simulink model "pmsmfoc_cleaned"  (R2022b)
settings: Solver=ode1  StartTime=0.0  StopTime=0.2  FixedStep=ctrlConst.TsSwitch  MaxStep=1e-6  RelTol=1e-3  EnableMultiTasking=on
PreLoadFcn:
  | %rtwdemo_pmsmfoc_data
StartFcn:
  | %clear executionProfile
StopFcn:
  | %try
  | %  AddExecutionProfileToDataInspector();
  | %end
undefined symbols (not defined in the file): ECM, EGM, fsw, g_msgCore0to2_pwmFrqSet, g_msgCore0to2_SpeedType_Switch, PWMFrqSwitch_C, SC_Ld_P, SC_Lq_P, SC_Psi_P, SC_Rs20_P, Ts_10ms, Ts_1ms, Tsw
libraries: MathLib x3
(part 1 of 2)
settings Model: Creator=The MathWorks, Inc.  LastModifiedBy=HP
settings SolverCC: AlgebraicLoopSolver=TrustRegion  InsertRTBMode=Never (minimum delay)
settings DataIOCC: LimitDataPoints=on  SaveFormat=Array  SaveOutput=off  SaveTime=off
settings OptimizationCC: DefaultParameterBehavior=Inlined  UseDivisionForNetSlopeComputation=on  UseFloatMulNetSlope=on  DefaultUnderspecifiedDataType=single  InlineInvariantSignals=on  PassReuseOutputArgsAs=Individual arguments  ExpressionDepthLimit=2147483647  ZeroExternalMemoryAtStartup=off  ZeroInternalMemoryAtStartup=off  NoFixptDivByZeroProtection=on  EfficientFloat2IntCast=on  LifeSpan=1  EfficientTunableParamExpr=on
settings DebuggingCC: ReadBeforeWriteMsg=DisableAll  WriteAfterWriteMsg=DisableAll  WriteAfterReadMsg=DisableAll  AlgebraicLoopMsg=none  MultiTaskDSMMsg=none  SingleTaskRateTransMsg=error  IntegerOverflowMsg=none  ParameterPrecisionLossMsg=none  BusObjectLabelMismatch=none  AssertControl=DisableAll  AllowSymbolicDim=off  StateNameClashWarn=warning  SFUnexpectedBacktrackingDiag=warning  SFNoUnconditionalDefaultTransitionDiag=warning  SFExecutionAtInitializationDiag=none  SFMachineParentedDataDiag=warning  IntegerSaturationMsg=none  UnitsInconsistencyMsg=none  ArithmeticOperatorsInVariantConditions=warning
settings HardwareCC: ProdBitPerPointer=32  ProdBitPerSizeT=32  ProdBitPerPtrDiffT=32  ProdLargestAtomicFloat=None  ProdWordSize=32  ProdHWDeviceType=Infineon->TriCore
settings ModelReferenceCC: UpdateModelReferenceTargets=IfOutOfDate  EnableRefExpFcnMdlSchedulingChecks=on  ModelReferenceNumInstancesAllowed=Single  PropagateSignalLabelsOutOfModel=off
settings SFSimCC: SFSimEcho=off  SimUseLocalCustomCode=off  SimGenImportedTypeDefs=on  MATLABDynamicMemAlloc=off  CustomCodeUndefinedFunction=UseInterfaceOnly
settings RTWCC: Description=Embedded Coder  SystemTargetFile=ert.tlc  GenCodeOnly=on  GenerateMakefile=off  TemplateMakefile=ec_target.tmf  RTWVerbose=off  RTWUseLocalCustomCode=off  CodeExecutionProfiling=on  CodeProfilingSaveOptions=AllData  CodeProfilingInstrumentation=detailed
settings CodeAppCC: ForceParamTrailComments=on  IgnoreCustomStorageClasses=off  IgnoreTestpoints=on  MaxIdLength=64  SimulinkDataObjDesc=on  MATLABFcnDesc=on  CustomSymbolStrGlobalVar=GR$N$M  CustomSymbolStrType=pmsmfoc_$N$M  CustomSymbolStrFcn=$N$M$F  CustomSymbolStrFcnArg=$I$N$M  CustomSymbolStrMacro=$N$M  InsertBlockDesc=on  StateflowObjectComments=on  MATLABSourceComments=on  InternalIdentifier=Classic
settings ERTTargetCC: TargetLangStandard=C99 (ISO)  UtilityFuncGeneration=Shared location  MultiwordLength=2048  CombineSignalStateStructs=on  SupportAbsoluteTime=off  SupportNonFinite=off  SupportComplex=off  SupportNonInlinedSFcns=on  RemoveResetFunc=off  ParenthesesLevel=Maximum  GenerateASAP2=on  InlinedParameterPlacement=NonHierarchical  ERTCustomFileTemplate=example_file_process.tlc  EnableDataOwnership=on  ConvertIfToSwitch=off  SuppressUnreachableDefaultCases=off  MemSecPackage=Simulink  MemSecDataConstants=MemConst  MemSecDataParameters=MemConstVolatile
settings ConfigComp: CovMetricSettings=dcmtrzow  CovHTMLOptions=-aTS=1 -bRG=1 -bTC=1 -hTR=0 -nFC=0 -scm=1 -bcm=1 -xEv=0  CovSaveCumulativeToWorkspaceVar=on  CovSaveSingleToWorkspaceVar=on  CovExternalEMLEnable=off  CovSFcnEnable=off
settings SimscapeCC: SimscapeNormalizeSystem=off

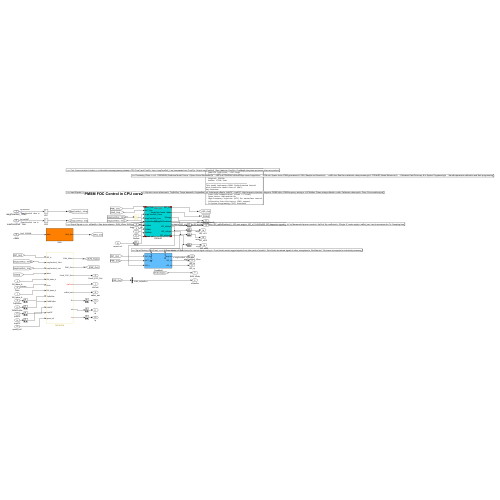
[thumbnail: Simulink's stored preview of the top-level diagram]
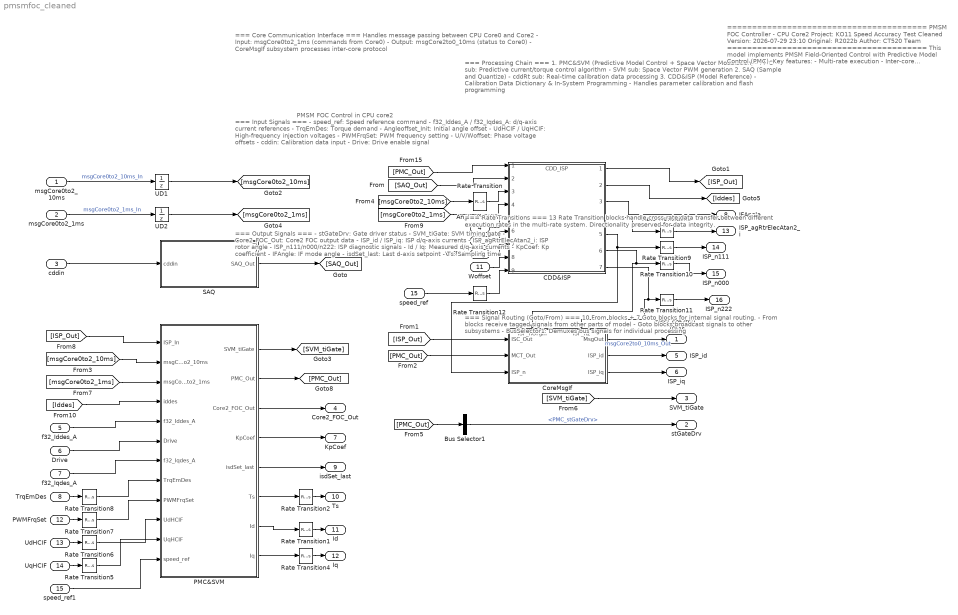
== system pmsmfoc_cleaned ==
  note: PMSM FOC Control in CPU core2
  note: === Core Communication Interface ===\nHandles message passing between CPU Core0 and Core2\n- Input: msgCore0to2_1ms (commands from Core0)\n- Output: msgCore2to0_10ms (status to Core0)\n- CoreMsgIf subsystem processes inter-core protocol
  note: === Input Signals ===\n- speed_ref: Speed reference command\n- f32_Iddes_A / f32_Iqdes_A: d/q-axis current references\n- TrqEmDes: Torque demand\n- Angleoffset_Init: Initial angle offset\n- UdHCIF / UqHCIF: High-frequency injection voltages\n- PWMFrqSet: PWM frequency setting\n- U/V/Woffset: Phase voltage offsets\n- cddin: Calibration data input\n- Drive: Drive enable signal
  note: === Output Signals ===\n- stGateDrv: Gate driver status\n- SVM_tiGate: SVM timing gate\n- Core2_FOC_Out: Core2 FOC output data\n- ISP_id / ISP_iq: ISP d/q-axis currents\n- ISP_agRtrElecAtan2_i: ISP rotor angle\n- ISP_n111/n000/n222: ISP diagnostic signals\n- Id / Iq: Measured d/q-axis currents\n- KpCoef: Kp coefficient\n- IFAngle: IF mode angle\n- isdSet_last: Last d-axis setpoint\n- Ts: Sampling time
  note: === Processing Chain ===\n1. PMC&SVM (Predictive Model Control + Space Vector Modulation)\n - PMC sub: Predictive current/torque control algorithm\n - SVM sub: Space Vector PWM generation\n2. SAQ (Sample and Quantize)\n - cddRt sub: Real-time calibration data processing\n3. CDD&ISP (Model Reference)\n - Calibration Data Dictionary & In-System Programming\n - Handles parameter calibration and flash programming
  note: === Rate Transitions ===\n13 Rate Transition blocks handle cross-rate data transfer\nbetween different execution rates in the multi-rate system.\nDirectionality preserved for data integrity.
  note: === Signal Routing (Goto/From) ===\n10 From blocks + 7 Goto blocks for internal signal routing.\n- From blocks receive tagged signals from other parts of model\n- Goto blocks broadcast signals to other subsystems\n- BusSelector1: Demuxes bus signals for individual processing
  note: ========================================
      |   PMSM FOC Controller - CPU Core2
      |   Project: KO11 Speed Accuracy Test
      |   Cleaned Version: 2026-07-29 23:10
      |   Original: R2022b
      |   Author: CT520 Team
      | ========================================
      | This model implements PMSM Field-Oriented Control
      | with Predictive Model Control (PMC).
      | Key features:
      | - Multi-rate execution
      | - Inter-core communication (Core0 <-> Core2)
      | - Space Vector PWM modulation
      | - High-Frequency Injection (HFI) for sensorless control
      | - Calibration Data Dictionary (CDD) support
      | - In-System Programming (ISP) interface
  msgCore0to2_10ms : Inport  OutDataTypeStr=Bus: Sig10ms02ST  SampleTime=Ts_1ms  BusOutputAsStruct=on
  msgCore0to2_1ms : Inport  Port=2  OutDataTypeStr=Bus: Sig1ms02ST  SampleTime=Ts_1ms  BusOutputAsStruct=on
  cddin : Inport  Port=3  OutDataTypeStr=Bus: Core2_CDDIN2  SampleTime=Tsw  BusOutputAsStruct=on
  Angleoffset_Init : Inport  Port=4  OutDataTypeStr=int16  SampleTime=Ts_10ms
  f32_Iddes_A : Inport  Port=5
  Drive : Inport  Port=6  OutDataTypeStr=boolean
  f32_Iqdes_A : Inport  Port=7
  TrqEmDes : Inport  Port=8
  Uoffset : Inport  Port=9
  Voffset : Inport  Port=10
  Woffset : Inport  Port=11
  PWMFrqSet : Inport  Port=12
  UdHCIF : Inport  Port=13
  UqHCIF : Inport  Port=14
  speed_ref : Inport  Port=15
  Bus Selector1 : BusSelector  OutputSignals=PMC_stGateDrv
  CDD&ISP : ModelReference  ModelNameDialog=CDD_ISP.slx  SimulationMode=Normal  ModelReferenceVersion=1.237
  CoreMsgIf : Subsystem
      settings: PortSchema="{\"entries\":[{\"content\":{\"sides\":[{\"content\":{\"connectorIds\":[\"In1\",\"In2\",\"In3\"]},\"type\":\"ConnectorPlacement.EquallySpacedRectSide\",\"uuid\":\"1bc9449b-5392-4ed5-810c-ef0b1f3a3873\"},{\"content\":{\"connectorIds\":[\"Out1\",\"Out2\",\"Out3\"],\"side\":\"RIGHT\"},\"type\":\"ConnectorPlacement.EquallySpacedRectSide\",\"uuid\":\"ebce0c42-110a-49f6-97c9-7794c95f763f\"},{\"content\":{\"connectorIds\":[\"In4\",\"In5\"],\"side\":\"TOP\"},\"type\":\"ConnectorPlacement.EquallySpacedRectSide\",\"uuid\":\"d14212b0-cf9d-44fe-a2d1-1375008f2372\"}]},\"type\":\"ConnectorPlacement.EquallySpacedConnector\",\"uuid\":\"c8a2bb93-ddbf-4abc-bd38-97ecc81d6200\"}],\"packageUris\":[\"http://schema.mathworks.com/mf0/Connector/R2020b\"],\"version\":\"1.0\"}"
  PMC&SVM : Subsystem  RequirementInfo={} %GIDa_aba5f94c_bdce_4442_83f7_df5d7516f2fa
      settings: MinAlgLoopOccurrences=on
  Rate Transition : RateTransition  Deterministic=off
  Rate Transition{1..2,4..8,12} (8 alike) : RateTransition  Deterministic=off  InitialCondition=ECM.Init
  Rate Transition{3,9..11} (4 alike) : RateTransition
  SAQ : Subsystem
  UD1 : UnitDelay  SampleTime=-1  HasFrameUpgradeWarning=on
  UD2 : UnitDelay  SampleTime=-1  HasFrameUpgradeWarning=on
  speed_ref1 : InportShadow  Port=15
  msgCore2to0_10ms : Outport  OutDataTypeStr=Bus: Sig10ms20ST  VectorParamsAs1DForOutWhenUnconnected=off
  stGateDrv : Outport  Port=2  VectorParamsAs1DForOutWhenUnconnected=off
  SVM_tiGate : Outport  Port=3  VectorParamsAs1DForOutWhenUnconnected=off
  Core2_FOC_Out : Outport  Port=4
  ISP_id : Outport  Port=5
  ISP_iq : Outport  Port=6
  KpCoef : Outport  Port=7
  IFAngle : Outport  Port=8
  isdSet_last : Outport  Port=9
  Ts : Outport  Port=10
  Id : Outport  Port=11
  Iq : Outport  Port=12
  ISP_agRtrElecAtan2_i : Outport  Port=13
  ISP_n111 : Outport  Port=14  OutDataTypeStr=single
  ISP_n000 : Outport  Port=15  OutDataTypeStr=single
  ISP_n222 : Outport  Port=16  OutDataTypeStr=single
  wires:
  cddin/1 -> SAQ/1(cddin)
  SAQ/1(SAQ_Out) -> [SAQ_Out]
  [SAQ_Out] -> CDD&ISP/2
  CDD&ISP/1 -> [ISP_Out]
  [ISP_Out] -> PMC&SVM/1(ISP_In)
  [PMC_Out] -> CDD&ISP/1
  Bus Selector1/1 -> stGateDrv/1  "<PMC_stGateDrv>"
  [msgCore0to2_10ms] -> PMC&SVM/2(msgCore0to2_10ms)
  msgCore0to2_1ms/1 -> UD2/1  "msgCore0to2_1ms_In"
  [msgCore0to2_10ms] -> Rate Transition/1
  [ISP_Out] -> CoreMsgIf/1(ISC_Out)
  [PMC_Out] -> CoreMsgIf/2(MCT_Out)
  [PMC_Out] -> Bus Selector1/1
  [SVM_tiGate] -> SVM_tiGate/1
  CoreMsgIf/1(MsgOut) -> msgCore2to0_10ms/1  "msgCore2to0_10ms_Out"
  msgCore0to2_10ms/1 -> UD1/1  "msgCore0to2_10ms_In"
  UD1/1 -> [msgCore0to2_10ms]
  [msgCore0to2_1ms] -> PMC&SVM/3(msgCore0to2_1ms)
  UD2/1 -> [msgCore0to2_1ms]
  [msgCore0to2_1ms] -> CDD&ISP/4
  PMC&SVM/1(SVM_tiGate) -> [SVM_tiGate]
  PMC&SVM/2(PMC_Out) -> [PMC_Out]
  Rate Transition/1 -> CDD&ISP/3
  PMC&SVM/3(Core2_FOC_Out) -> Core2_FOC_Out/1
  CoreMsgIf/2(ISP_id) -> ISP_id/1
  CoreMsgIf/3(ISP_iq) -> ISP_iq/1
  CDD&ISP/2 -> [Iddes]
  [Iddes] -> PMC&SVM/4(iddes)
  Angleoffset_Init/1 -> CDD&ISP/5
  f32_Iddes_A/1 -> PMC&SVM/5(f32_Iddes_A)
  Drive/1 -> PMC&SVM/6(Drive)
  f32_Iqdes_A/1 -> PMC&SVM/7(f32_Iqdes_A)
  PMC&SVM/4(KpCoef) -> KpCoef/1
  TrqEmDes/1 -> Rate Transition8/1
  PMC&SVM/5(isdSet_last) -> isdSet_last/1
  PMC&SVM/6(Ts) -> Rate Transition2/1
  PMC&SVM/7(Id) -> Rate Transition1/1
  PMC&SVM/8(Iq) -> Rate Transition4/1
  Uoffset/1 -> CDD&ISP/6
  Voffset/1 -> CDD&ISP/7
  Woffset/1 -> CDD&ISP/8
  PWMFrqSet/1 -> Rate Transition7/1
  Rate Transition4/1 -> Iq/1
  Rate Transition1/1 -> Id/1
  Rate Transition2/1 -> Ts/1
  UdHCIF/1 -> Rate Transition6/1
  UqHCIF/1 -> Rate Transition5/1
  CDD&ISP/3 -> IFAngle/1
  CDD&ISP/4 -> Rate Transition3/1
  Rate Transition3/1 -> ISP_agRtrElecAtan2_i/1
  Rate Transition5/1 -> PMC&SVM/11(UqHCIF)
  Rate Transition6/1 -> PMC&SVM/10(UdHCIF)
  Rate Transition7/1 -> PMC&SVM/9(PWMFrqSet)
  Rate Transition8/1 -> PMC&SVM/8(TrqEmDes)
  CDD&ISP/5 -> Rate Transition9/1, CoreMsgIf/3(ISP_n)
  Rate Transition9/1 -> ISP_n111/1
  CDD&ISP/6 -> Rate Transition10/1, CoreMsgIf/4(ISP_nOrgin)
  Rate Transition10/1 -> ISP_n000/1
  speed_ref/1 -> Rate Transition12/1
  Rate Transition12/1 -> CDD&ISP/9
  Rate Transition11/1 -> ISP_n222/1
  CDD&ISP/7 -> Rate Transition11/1, CoreMsgIf/5(ISP_n2)
  speed_ref1/1 -> PMC&SVM/12(speed_ref)

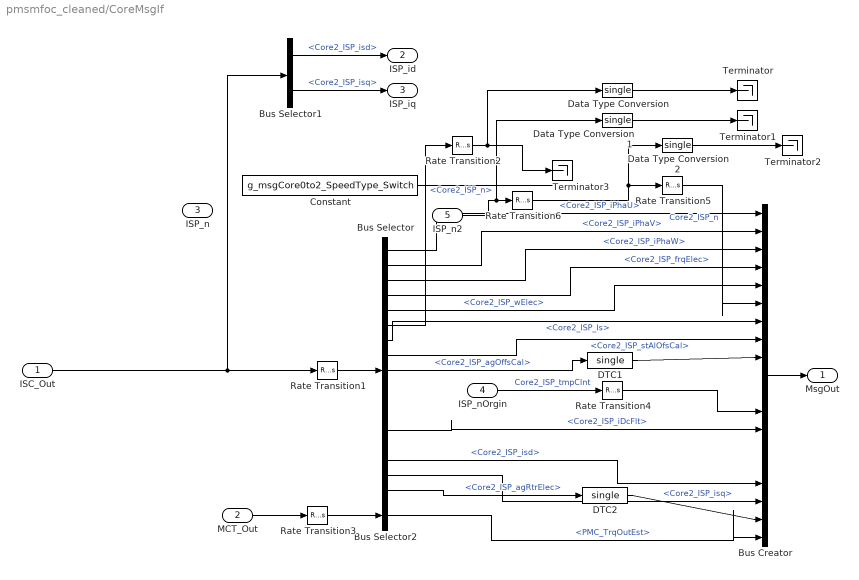
== system pmsmfoc_cleaned/CoreMsgIf ==
  ISC_Out : Inport  OutDataTypeStr=Bus: Core2_ISP_Out
  MCT_Out : Inport  Port=2
  ISP_n : Inport  Port=3
  ISP_nOrgin : Inport  Port=4
  ISP_n2 : Inport  Port=5
  Bus Creator : BusCreator  Inputs=19  OutDataTypeStr=Bus:Sig10ms20ST  NonVirtualBus=on
      settings: InheritFromInputs=off
  Bus Selector : BusSelector  OutputSignals=Core2_ISP_AnaOut.Core2_ISP_iPhabc.Core2_ISP_iPhaU,Core2_ISP_AnaOut.Core2_ISP_iPhabc.Core2_ISP_iPhaV,Core2_ISP_AnaOut.Core2_ISP_iPhabc.Core2_ISP_iPhaW,Core2_ISP_nx.Core2_ISP_frqElec,Core2_ISP_nx.Core2_ISP_wElec,Core2_ISP_nx.Core2_ISP_n,Core2_ISP_Isx.Core2_ISP_Is,Core2_ISP_nx.Core2_ISP_stAlOfsCal,Core2_ISP_nx.Core2_ISP_agOffsCal,Core2_ISC_tmpOut.Core2_ISP_tmpMaxIGBT,Core2_ISC_tmpOut.Core2_ISP_tmpClnt,Core2_ISC_tmpOut.Core2_ISP_lossTotalIGBT,Core2_ISC_tmpOut.Core2_ISP_iDcFlt,Core2_ISP_AnaOut.Core2_ISP_bIphCalDone,Core2_ISP_Isx.Core2_ISP_isd,Core2_ISP_Isx.Core2_ISP_isq,Core2_ISP_nx.Core2_ISP_agRtrElec
  Bus Selector1 : BusSelector  OutputSignals=Core2_ISP_Isx.Core2_ISP_isd,Core2_ISP_Isx.Core2_ISP_isq
  Bus Selector2 : BusSelector  OutputSignals=PMC_TrqOutEst
  Constant : Constant  Value=g_msgCore0to2_SpeedType_Switch
  DTC1 : DataTypeConversion  OutDataTypeStr=single  SaturateOnIntegerOverflow=off  RndMeth=Floor
  DTC2 : DataTypeConversion  OutDataTypeStr=single  SaturateOnIntegerOverflow=off  RndMeth=Floor
  Data Type Conversion : DataTypeConversion  OutDataTypeStr=single  SaturateOnIntegerOverflow=off  RndMeth=Floor
  Data Type Conversion1 : DataTypeConversion  OutDataTypeStr=single  SaturateOnIntegerOverflow=off  RndMeth=Floor
  Data Type Conversion2 : DataTypeConversion  OutDataTypeStr=single  SaturateOnIntegerOverflow=off  RndMeth=Floor
  Rate Transition{1..6} (6 alike) : RateTransition  Deterministic=off  OutPortSampleTime=Ts_1ms
  Terminator{,1..3} (4 alike) : Terminator
  MsgOut : Outport  OutDataTypeStr=Bus: Sig10ms20ST  VectorParamsAs1DForOutWhenUnconnected=off
  ISP_id : Outport  Port=2
  ISP_iq : Outport  Port=3
  wires:
  MCT_Out/1 -> Rate Transition3/1
  Rate Transition3/1 -> Bus Selector2/1
  Bus Selector/13 -> Bus Creator/13  "<Core2_ISP_iDcFlt>"
  ISC_Out/1 -> Rate Transition1/1, Bus Selector1/1
  Rate Transition1/1 -> Bus Selector/1
  Bus Selector/5 -> Bus Creator/5  "<Core2_ISP_wElec>"
  Bus Selector/4 -> Bus Creator/4  "<Core2_ISP_frqElec>"
  Bus Creator/1 -> MsgOut/1
  Bus Selector/7 -> Bus Creator/7  "<Core2_ISP_Is>"
  Bus Selector/8 -> Bus Creator/8  "<Core2_ISP_stAlOfsCal>"
  Bus Selector/9 -> DTC1/1  "<Core2_ISP_agOffsCal>"
  DTC1/1 -> Bus Creator/9
  Bus Selector/17 -> DTC2/1  "<Core2_ISP_agRtrElec>"
  Bus Selector/16 -> Bus Creator/17  "<Core2_ISP_isq>"
  Bus Selector/15 -> Bus Creator/16  "<Core2_ISP_isd>"
  DTC2/1 -> Bus Creator/18
  Bus Selector2/1 -> Bus Creator/19  "<PMC_TrqOutEst>"
  Bus Selector1/1 -> ISP_id/1  "<Core2_ISP_isd>"
  Bus Selector1/2 -> ISP_iq/1  "<Core2_ISP_isq>"
  Bus Selector/3 -> Bus Creator/3  "<Core2_ISP_iPhaW>"
  Bus Selector/2 -> Bus Creator/2  "<Core2_ISP_iPhaV>"
  Bus Selector/1 -> Bus Creator/1  "<Core2_ISP_iPhaU>"
  Rate Transition4/1 -> Bus Creator/12
  ISP_nOrgin/1 -> Rate Transition4/1  "Core2_ISP_tmpClnt"
  Bus Selector/6 -> Rate Transition2/1  "<Core2_ISP_n>"
  Rate Transition6/1 -> Data Type Conversion2/1, Rate Transition5/1
  ISP_n2/1 -> Data Type Conversion1/1, Rate Transition6/1
  Constant/1 -> ?
  Rate Transition2/1 -> Terminator3/1, Data Type Conversion/1
  Rate Transition5/1 -> Bus Creator/6  "Core2_ISP_n"
  Data Type Conversion/1 -> Terminator/1
  Data Type Conversion1/1 -> Terminator1/1
  Data Type Conversion2/1 -> Terminator2/1

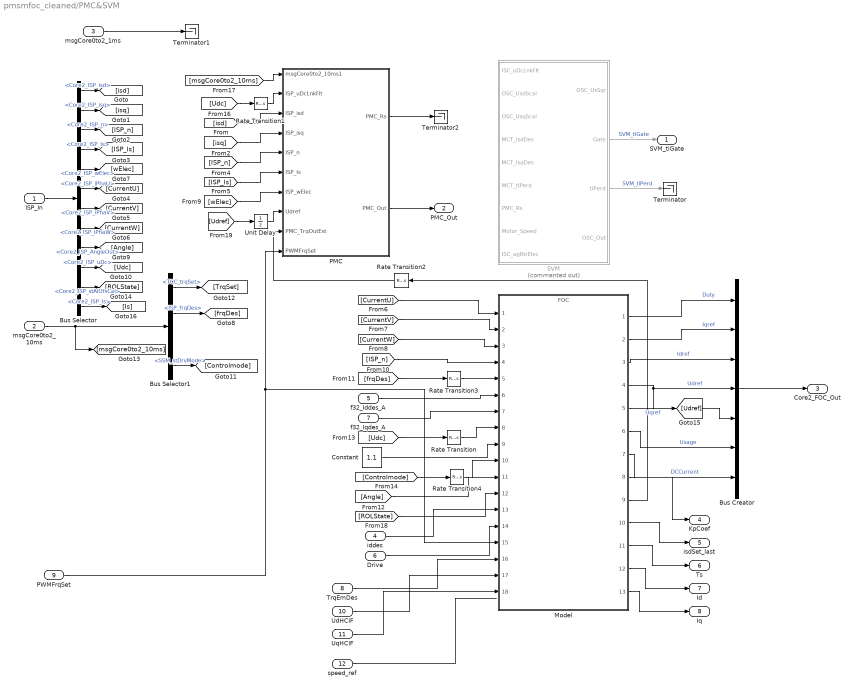
== system pmsmfoc_cleaned/PMC&SVM ==
  ISP_In : Inport  RequirementInfo={} %GIDa_f6540206_9371_47ef_bcdb_2ea40a07804d
  msgCore0to2_10ms : Inport  RequirementInfo={} %GIDa_db689c64_39e8_4f82_8312_263842f9e924  Port=2
  msgCore0to2_1ms : Inport  Port=3
  iddes : Inport  Port=4
  f32_Iddes_A : Inport  Port=5
  Drive : Inport  Port=6
  f32_Iqdes_A : Inport  Port=7
  TrqEmDes : Inport  Port=8
  PWMFrqSet : Inport  Port=9
  UdHCIF : Inport  Port=10
  UqHCIF : Inport  Port=11
  speed_ref : Inport  Port=12
  Bus Creator : BusCreator  Inputs=7  OutDataTypeStr=Bus: Core2_FOC_Out  NonVirtualBus=on
  Bus Selector : BusSelector  OutputSignals=Core2_ISP_Isx.Core2_ISP_isd,Core2_ISP_Isx.Core2_ISP_isq,Core2_ISP_nx.Core2_ISP_n,Core2_ISP_Isx.Core2_ISP_Is,Core2_ISP_nx.Core2_ISP_wElec,Core2_ISP_AnaOut.Core2_ISP_iPhabc.Core2_ISP_iPhaU,Core2_ISP_AnaOut.Core2_ISP_iPhabc.Core2_ISP_iPhaV,Core2_ISP_AnaOut.Core2_ISP_iPhabc.Core2_ISP_iPhaW,Core2_ISP_Isx.Core2_ISP_AngleOut,Core2_ISP_AnaOut.Core2_ISP_uDc,Core2_ISP_nx.Core2_ISP_stAlOfsCal,Core2_ISP_Isx.Core2_ISP_Is
  Bus Selector1 : BusSelector  OutputSignals=TCC_trqSet,ISP_frqDes,ISP_isDes,SSM_stDrvMode
  Constant : Constant  Value=1.1  OutDataTypeStr=single
  Model : ModelReference  ModelNameDialog=FOC.slx  SimulationMode=Normal  ModelReferenceVersion=1.230
  PMC : Subsystem  RequirementInfo={} %GIDa_45aea5b4_73b0_47d7_923a_5575377c0528  SystemSampleTime=Tsw
  Rate Transition{,1..3} (4 alike) : RateTransition  Deterministic=off
  Rate Transition4 : RateTransition  Deterministic=off  InitialCondition=ECM.Init
  SVM : Subsystem  Commented=on
  Terminator : Terminator
  Terminator1 : Terminator
  Terminator2 : Terminator
  Unit Delay : UnitDelay  SampleTime=-1  HasFrameUpgradeWarning=on
  SVM_tiGate : Outport  RequirementInfo={} %GIDa_247e6739_f09d_406d_b522_add8602f32ed  VectorParamsAs1DForOutWhenUnconnected=off
  PMC_Out : Outport  Port=2  OutDataTypeStr=Bus: Core2_PMC_Out  VectorParamsAs1DForOutWhenUnconnected=off
  Core2_FOC_Out : Outport  Port=3
  KpCoef : Outport  Port=4
  isdSet_last : Outport  Port=5
  Ts : Outport  Port=6
  Id : Outport  Port=7
  Iq : Outport  Port=8
  wires:
  SVM/2(Gate) -> SVM_tiGate/1  "SVM_tiGate"
  Rate Transition1/1 -> PMC/2(ISP_uDcLnkFlt)
  ISP_In/1 -> Bus Selector/1
  PMC/2(PMC_Out) -> PMC_Out/1
  msgCore0to2_10ms/1 -> Bus Selector1/1, [msgCore0to2_10ms]
  SVM/3(tiPerd) -> Terminator/1  "SVM_tiPerd"
  msgCore0to2_1ms/1 -> Terminator1/1
  PMC/1(PMC_Rs) -> Terminator2/1
  Constant/1 -> Model/9
  Rate Transition3/1 -> Model/5
  Rate Transition/1 -> Model/8
  Rate Transition4/1 -> Model/10
  Model/1 -> Bus Creator/1  "Duty"
  Model/2 -> Bus Creator/2  "Iqref"
  Model/3 -> Bus Creator/3  "Idref"
  Model/4 -> Bus Creator/4, [Udref]  "Udref"
  Model/5 -> Bus Creator/5  "Uqref"
  Bus Creator/1 -> Core2_FOC_Out/1
  Bus Selector/1 -> [isd]  "<Core2_ISP_isd>"
  [isd] -> PMC/3(ISP_isd)
  [isq] -> PMC/4(ISP_isq)
  Bus Selector/2 -> [isq]  "<Core2_ISP_isq>"
  Bus Selector/3 -> [ISP_n]  "<Core2_ISP_n>"
  [ISP_n] -> PMC/5(ISP_n)
  Bus Selector/4 -> [ISP_Is]  "<Core2_ISP_Is>"
  [ISP_Is] -> PMC/6(ISP_Is)
  Bus Selector/6 -> [CurrentU]  "<Core2_ISP_iPhaU>"
  Bus Selector/7 -> [CurrentV]  "<Core2_ISP_iPhaV>"
  Bus Selector/8 -> [CurrentW]  "<Core2_ISP_iPhaW>"
  [CurrentU] -> Model/1
  [CurrentV] -> Model/2
  [CurrentW] -> Model/3
  Bus Selector/5 -> [wElec]  "<Core2_ISP_wElec>"
  [wElec] -> PMC/7(ISP_wElec)
  [ISP_n] -> Model/4
  Bus Selector1/2 -> [frqDes]  "<ISP_frqDes>"
  [frqDes] -> Rate Transition3/1
  Bus Selector/9 -> [Angle]  "<Core2_ISP_AngleOut>"
  [Angle] -> Model/11
  Bus Selector/10 -> [Udc]  "<Core2_ISP_uDc>"
  [Udc] -> Rate Transition/1
  Bus Selector1/4 -> [Controlmode]  "<SSM_stDrvMode>"
  [Controlmode] -> Rate Transition4/1
  Bus Selector1/1 -> [TrqSet]  "<TCC_trqSet>"
  [Udc] -> Rate Transition1/1
  [msgCore0to2_10ms] -> PMC/1(msgCore0to2_10ms1)
  Bus Selector/11 -> [ROLState]  "<Core2_ISP_stAlOfsCal>"
  [ROLState] -> Model/12
  iddes/1 -> Model/13
  f32_Iddes_A/1 -> Model/6
  Drive/1 -> Model/14
  f32_Iqdes_A/1 -> Model/7
  [Udref] -> Unit Delay/1
  Unit Delay/1 -> PMC/8(Udref)
  Bus Selector/12 -> [Is]  "<Core2_ISP_Is>"
  Model/8 -> KpCoef/1
  Model/6 -> Bus Creator/6  "Usage"
  Model/7 -> Bus Creator/7  "DCCurrent"
  Model/9 -> Rate Transition2/1
  TrqEmDes/1 -> Model/16
  Model/10 -> isdSet_last/1
  Model/11 -> Ts/1
  Model/12 -> Id/1
  Model/13 -> Iq/1
  PWMFrqSet/1 -> PMC/10(PWMFrqSet), Model/15
  UdHCIF/1 -> Model/17
  UqHCIF/1 -> Model/18
  Rate Transition2/1 -> PMC/9(PMC_TrqOutEst)
  speed_ref/1 -> ?

== system pmsmfoc_cleaned/SAQ ==
  cddin : Inport
  cddRt : Subsystem
  SAQ_Out : Outport  OutDataTypeStr=Bus: Core2_SAQ_Out  VectorParamsAs1DForOutWhenUnconnected=off
      settings: AttributesFormatString=Disable Action: %<OutputWhenDisabled>
  wires:
  cddRt/1(cddSig) -> SAQ_Out/1  "cddRt"
  cddin/1 -> cddRt/1(cddSt)

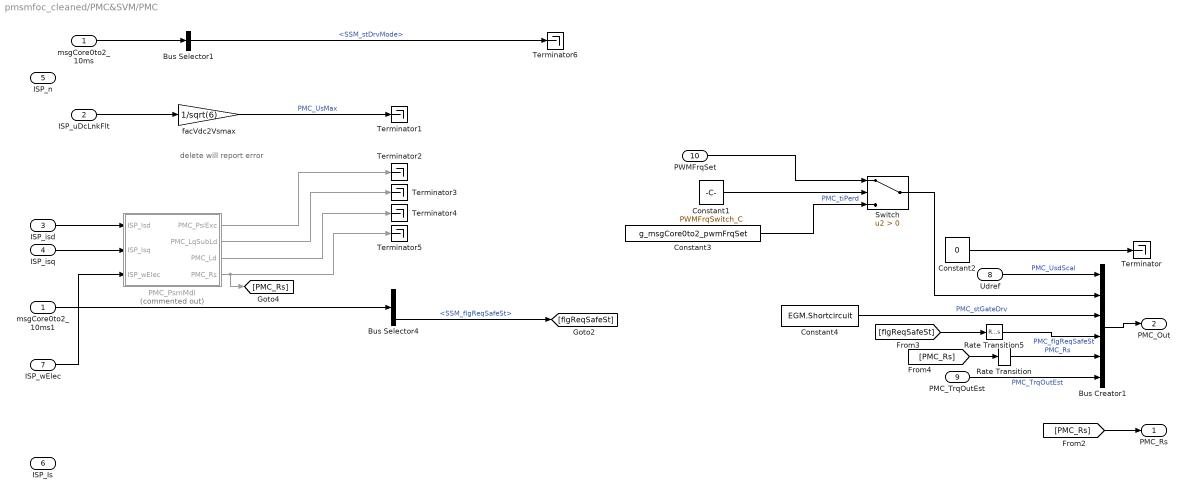
== system pmsmfoc_cleaned/PMC&SVM/PMC ==
  note: delete will report error
  msgCore0to2_10ms1 : Inport  RequirementInfo={} %GIDa_62968669_2ac2_4296_9b34_9acab11e3351
  ISP_uDcLnkFlt : Inport  RequirementInfo={} %GIDa_ca93117e_11ed_4a5d_b591_b702703c2b5a  Port=2
  ISP_isd : Inport  RequirementInfo={} %GIDa_4c76f347_a6a1_47a4_b7d0_60bec3ffd976  Port=3
  ISP_isq : Inport  RequirementInfo={} %GIDa_70459766_063a_410f_849e_470931a9729a  Port=4
  ISP_n : Inport  Port=5
  ISP_Is : Inport  Port=6
  ISP_wElec : Inport  RequirementInfo={} %GIDa_15028701_01af_406d_8077_8bad37e851e9  Port=7
  Udref : Inport  Port=8
  PMC_TrqOutEst : Inport  Port=9
  PWMFrqSet : Inport  Port=10
  Bus Creator1 : BusCreator  Inputs=6  OutDataTypeStr=Bus: Core2_PMC_Out  NonVirtualBus=on
  Bus Selector1 : BusSelector  OutputSignals=SSM_stDrvMode
  Bus Selector4 : BusSelector  OutputSignals=SSM_stGateDrv,SSM_stDrvMode,SSM_flgReqSafeSt
  Constant1 : Constant  Value=PWMFrqSwitch_C
  Constant2 : Constant  Value=0  OutDataTypeStr=single  SampleTime=-1
  Constant3 : Constant  Value=g_msgCore0to2_pwmFrqSet  OutDataTypeStr=single  SampleTime=-1
  Constant4 : Constant  Value=EGM.Shortcircuit  OutDataTypeStr=Enum: EGM
  PMC_PsmMdl : Subsystem  RequirementInfo={} %GIDa_c46a785d_0a8b_4cc8_8d66_3e5f2fce2378  Commented=on
  Rate Transition : RateTransition  Deterministic=off
  Rate Transition5 : RateTransition  Deterministic=off  OutPortSampleTime=Tsw
  Switch : Switch  Criteria=u2 > Threshold  SaturateOnIntegerOverflow=off  InputSameDT=off
  Terminator{,1..6} (7 alike) : Terminator
  facVdc2Vsmax : Gain  RequirementInfo={} %GIDa_223ddcfe_885a_4a4c_9204_a9c8c9b1baab  Gain=1/sqrt(6)
  msgCore0to2_10ms : InportShadow
  PMC_Rs : Outport  VectorParamsAs1DForOutWhenUnconnected=off
  PMC_Out : Outport  Port=2  OutDataTypeStr=Bus: Core2_PMC_Out  VectorParamsAs1DForOutWhenUnconnected=off
  wires:
  Constant2/1 -> Terminator/1
  Udref/1 -> Bus Creator1/1  "PMC_UsdScal"
  facVdc2Vsmax/1 -> Terminator1/1  "PMC_UsMax"
  ISP_wElec/1 -> PMC_PsmMdl/3(ISP_wElec)
  ISP_uDcLnkFlt/1 -> facVdc2Vsmax/1
  PMC_PsmMdl/3(PMC_Ld) -> Terminator4/1
  PMC_PsmMdl/2(PMC_LqSubLd) -> Terminator3/1
  PMC_PsmMdl/1(PMC_PsiExc) -> Terminator2/1
  msgCore0to2_10ms1/1 -> Bus Selector4/1
  ISP_isq/1 -> PMC_PsmMdl/2(ISP_Isq)
  ISP_isd/1 -> PMC_PsmMdl/1(ISP_Isd)
  Bus Creator1/1 -> PMC_Out/1
  Constant4/1 -> Bus Creator1/3  "PMC_stGateDrv"
  Bus Selector4/3 -> [flgReqSafeSt]  "<SSM_flgReqSafeSt>"
  Rate Transition5/1 -> Bus Creator1/4  "PMC_flgReqSafeSt"
  Constant3/1 -> Switch/3  "PMC_tiPerd"
  PMC_PsmMdl/4(PMC_Rs) -> Terminator5/1, [PMC_Rs]
  [flgReqSafeSt] -> Rate Transition5/1
  [PMC_Rs] -> Rate Transition/1
  msgCore0to2_10ms/1 -> Bus Selector1/1
  Bus Selector1/1 -> Terminator6/1  "<SSM_stDrvMode>"
  [PMC_Rs] -> PMC_Rs/1
  Rate Transition/1 -> Bus Creator1/5  "PMC_Rs"
  PMC_TrqOutEst/1 -> Bus Creator1/6  "PMC_TrqOutEst"
  Constant1/1 -> Switch/2
  PWMFrqSet/1 -> Switch/1
  Switch/1 -> Bus Creator1/2

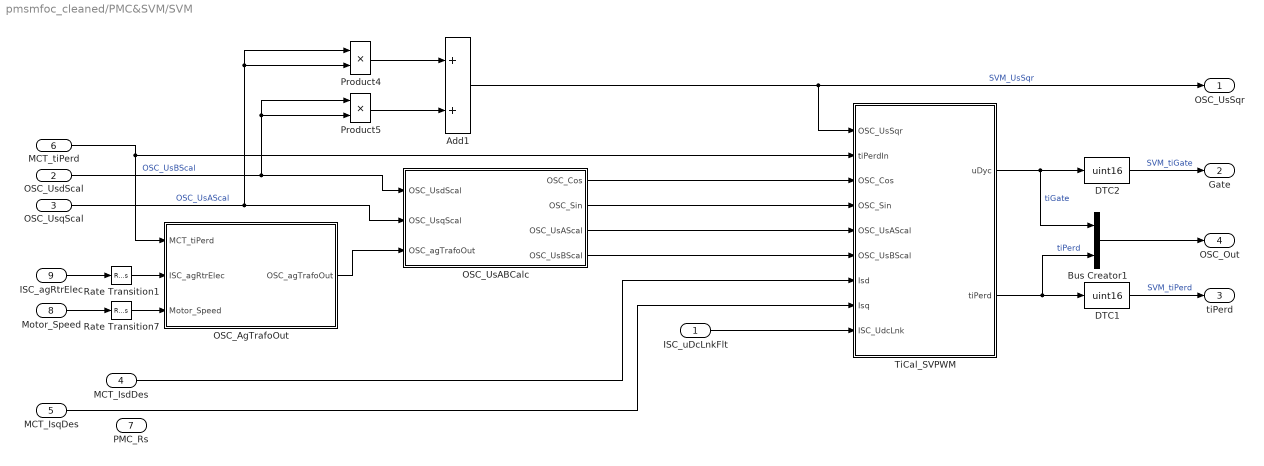
== system pmsmfoc_cleaned/PMC&SVM/SVM ==
  ISC_uDcLnkFlt : Inport
  OSC_UsdScal : Inport  Port=2
  OSC_UsqScal : Inport  Port=3
  MCT_IsdDes : Inport  Port=4
  MCT_IsqDes : Inport  Port=5
  MCT_tiPerd : Inport  Port=6
  PMC_Rs : Inport  Port=7
  Motor_Speed : Inport  Port=8
  ISC_agRtrElec : Inport  Port=9
  Add1 : Sum
  Bus Creator1 : BusCreator  Inputs=2
  DTC1 : DataTypeConversion  OutDataTypeStr=uint16  ConvertRealWorld=Stored Integer (SI)  RndMeth=Floor
  DTC2 : DataTypeConversion  OutDataTypeStr=uint16  ConvertRealWorld=Stored Integer (SI)  RndMeth=Floor
  OSC_AgTrafoOut : Subsystem  SystemSampleTime=1/fsw
  OSC_UsABCalc : Subsystem  SystemSampleTime=1/fsw
  Product4 : Product  RndMeth=Zero
  Product5 : Product  RndMeth=Zero
  Rate Transition1 : RateTransition  OutPortSampleTime=Tsw
  Rate Transition7 : RateTransition  OutPortSampleTime=Tsw
  TiCal_SVPWM : Subsystem  SystemSampleTime=1/fsw
  OSC_UsSqr : Outport  VectorParamsAs1DForOutWhenUnconnected=off
  Gate : Outport  Port=2  VectorParamsAs1DForOutWhenUnconnected=off
  tiPerd : Outport  Port=3  VectorParamsAs1DForOutWhenUnconnected=off
  OSC_Out : Outport  Port=4  VectorParamsAs1DForOutWhenUnconnected=off
  wires:
  DTC1/1 -> tiPerd/1  "SVM_tiPerd"
  Rate Transition1/1 -> OSC_AgTrafoOut/2(ISC_agRtrElec)
  DTC2/1 -> Gate/1  "SVM_tiGate"
  OSC_UsABCalc/1(OSC_Cos) -> TiCal_SVPWM/3(OSC_Cos)
  OSC_UsABCalc/2(OSC_Sin) -> TiCal_SVPWM/4(OSC_Sin)
  OSC_UsABCalc/4(OSC_UsBScal) -> TiCal_SVPWM/6(OSC_UsBScal)
  OSC_UsABCalc/3(OSC_UsAScal) -> TiCal_SVPWM/5(OSC_UsAScal)
  Rate Transition7/1 -> OSC_AgTrafoOut/3(Motor_Speed)
  Motor_Speed/1 -> Rate Transition7/1
  ISC_agRtrElec/1 -> Rate Transition1/1
  Bus Creator1/1 -> OSC_Out/1
  OSC_AgTrafoOut/1(OSC_agTrafoOut) -> OSC_UsABCalc/3(OSC_agTrafoOut)
  ISC_uDcLnkFlt/1 -> TiCal_SVPWM/9(ISC_UdcLnk)
  MCT_IsdDes/1 -> TiCal_SVPWM/7(Isd)
  MCT_IsqDes/1 -> TiCal_SVPWM/8(Isq)
  TiCal_SVPWM/1(uDyc) -> Bus Creator1/1, DTC2/1  "tiGate"
  TiCal_SVPWM/2(tiPerd) -> Bus Creator1/2, DTC1/1  "tiPerd"
  MCT_tiPerd/1 -> TiCal_SVPWM/2(tiPerdIn), OSC_AgTrafoOut/1(MCT_tiPerd)
  Add1/1 -> TiCal_SVPWM/1(OSC_UsSqr), OSC_UsSqr/1  "SVM_UsSqr"
  Product4/1 -> Add1/1
  Product5/1 -> Add1/2
  OSC_UsdScal/1 -> OSC_UsABCalc/1(OSC_UsdScal), Product5/2, Product5/1  "OSC_UsBScal"
  OSC_UsqScal/1 -> OSC_UsABCalc/2(OSC_UsqScal), Product4/1, Product4/2  "OSC_UsAScal"

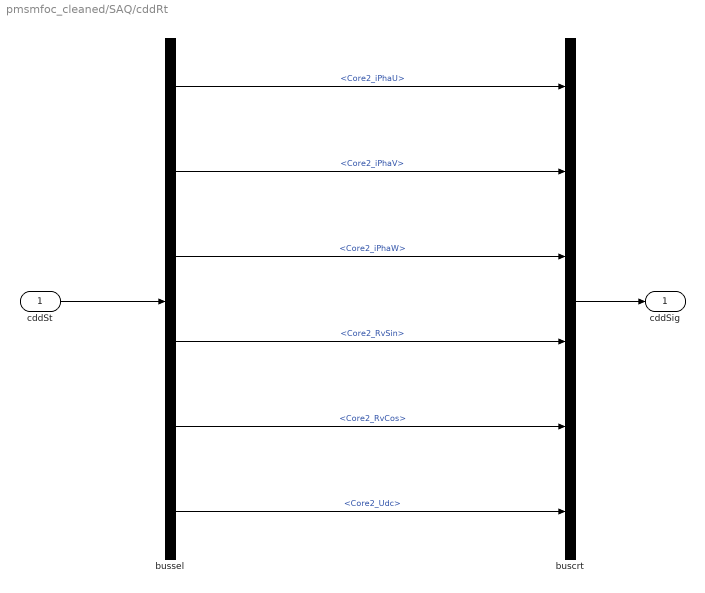
== system pmsmfoc_cleaned/SAQ/cddRt ==
  cddSt : Inport
  buscrt : BusCreator  Inputs=6  OutDataTypeStr=Bus: Core2_SAQ_Out
  bussel : BusSelector  OutputSignals=Core2_iPhaU,Core2_iPhaV,Core2_iPhaW,Core2_RvSin,Core2_RvCos,Core2_Udc
  cddSig : Outport  OutDataTypeStr=Bus: Core2_SAQ_Out
  wires:
  cddSt/1 -> bussel/1
  buscrt/1 -> cddSig/1
  bussel/1 -> buscrt/1  "<Core2_iPhaU>"
  bussel/2 -> buscrt/2  "<Core2_iPhaV>"
  bussel/3 -> buscrt/3  "<Core2_iPhaW>"
  bussel/4 -> buscrt/4  "<Core2_RvSin>"
  bussel/5 -> buscrt/5  "<Core2_RvCos>"
  bussel/6 -> buscrt/6  "<Core2_Udc>"

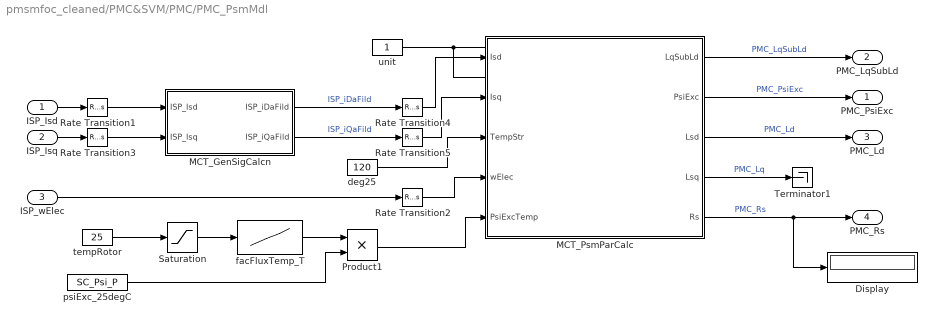
== system pmsmfoc_cleaned/PMC&SVM/PMC/PMC_PsmMdl ==
  ISP_Isd : Inport  RequirementInfo={} %GIDa_8af88909_b8c9_44df_9575_6eb027429994
  ISP_Isq : Inport  RequirementInfo={} %GIDa_ffb700a5_a8de_499d_94e7_08b94500e451  Port=2
  ISP_wElec : Inport  Port=3
  Display : Display
  MCT_GenSigCalcn : Subsystem  RequirementInfo={} %GIDa_627413f7_c9ac_4085_9ea5_ae65f1400bc9
  MCT_PsmParCalc : Subsystem  RequirementInfo={} %GIDa_4ca6e5ee_d847_4600_975d_35c05bb503c2  TreatAsAtomicUnit=on  SystemSampleTime=Ts_1ms
  Product1 : Product  OutDataTypeStr=single  RndMeth=Zero
  Rate Transition1 : RateTransition  RequirementInfo={} %GIDa_908af388_ca8c_4583_837c_1ab93633918a  Deterministic=off  OutPortSampleTime=Tsw
  Rate Transition2 : RateTransition  Deterministic=off  OutPortSampleTime=Ts_1ms
  Rate Transition3 : RateTransition  RequirementInfo={} %GIDa_5d4f7061_e977_434f_ae4e_c67ce52b6bf3  Deterministic=off  OutPortSampleTime=Tsw
  Rate Transition4 : RateTransition  RequirementInfo={} %GIDa_04c99b55_e048_4508_a917_2e4ff066b3c4  Deterministic=off  OutPortSampleTime=Ts_1ms
  Rate Transition5 : RateTransition  RequirementInfo={} %GIDa_c579dd9e_b002_4682_917a_cfeece666c4a  Deterministic=off  OutPortSampleTime=Ts_1ms
  Saturation : Saturate  UpperLimit=180  LowerLimit=-40
  Terminator1 : Terminator
      settings: RequirementInfo={} %GIDa_7b7a8826_de52_47d8_bb0c_199d9c94e2f6
  deg25 : Constant  RequirementInfo={} %GIDa_a4c3314b_7b34_4021_956b_a6c806554d01  Value=120  OutDataTypeStr=single  SampleTime=Ts_1ms
  facFluxTemp_T : Lookup_n-D  NumberOfTableDimensions=1  DataSpecification=Lookup table object  LookupTableObject=facFluxTemp_T  BreakpointsForDimension1="[0\t50\t100\t150\t200\t250\t300\t350\t400\t450       500]"  BeginIndexSearchUsingPreviousIndexResult=on  Table=|  ExtrapMethod=Clip  UseLastTableValue=on  InternalRulePriority=Speed  OutDataTypeStr=Inherit: Inherit from 'Table data'
      | [1	0.997426471	0.978676471	0.943382353	0.908823529	0.878676471	0.85	0.822794118	0.796139706	0.771691176	0.771507353
      | ]
  psiExc_25degC : Constant  Value=SC_Psi_P  OutDataTypeStr=single  SampleTime=Ts_1ms
  tempRotor : Constant  Value=25  OutDataTypeStr=single  SampleTime=Ts_1ms
  unit : Constant  RequirementInfo={} %GIDa_62859196_8da7_4c85_90d7_ef1ba9fdecfd  OutDataTypeStr=uint8  SampleTime=Ts_1ms
  PMC_PsiExc : Outport  RequirementInfo={} %GIDa_da38bff8_1d2a_41de_9c26_911309ad7c53  VectorParamsAs1DForOutWhenUnconnected=off
  PMC_LqSubLd : Outport  RequirementInfo={} %GIDa_e9d03f72_482c_45f8_bce9_a1bf1587484e  Port=2  VectorParamsAs1DForOutWhenUnconnected=off
  PMC_Ld : Outport  RequirementInfo={} %GIDa_5057aa34_b518_4703_9332_9b3e9fd72caa  Port=3  VectorParamsAs1DForOutWhenUnconnected=off
  PMC_Rs : Outport  Port=4  VectorParamsAs1DForOutWhenUnconnected=off
  wires:
  MCT_PsmParCalc/5(Rs) -> Display/1, PMC_Rs/1  "PMC_Rs"
  MCT_PsmParCalc/1(LqSubLd) -> PMC_LqSubLd/1  "PMC_LqSubLd"
  MCT_PsmParCalc/2(PsiExc) -> PMC_PsiExc/1  "PMC_PsiExc"
  Rate Transition5/1 -> MCT_PsmParCalc/2(Isq)
  Rate Transition4/1 -> MCT_PsmParCalc/1(Isd)
  Rate Transition3/1 -> MCT_GenSigCalcn/2(ISP_Isq)
  Rate Transition1/1 -> MCT_GenSigCalcn/1(ISP_Isd)
  MCT_GenSigCalcn/1(ISP_iDaFild) -> Rate Transition4/1  "ISP_iDaFild"
  ISP_Isq/1 -> Rate Transition3/1
  ISP_Isd/1 -> Rate Transition1/1
  MCT_GenSigCalcn/2(ISP_iQaFild) -> Rate Transition5/1  "ISP_iQaFild"
  MCT_PsmParCalc/3(Lsd) -> PMC_Ld/1  "PMC_Ld"
  MCT_PsmParCalc/4(Lsq) -> Terminator1/1  "PMC_Lq"
  deg25/1 -> MCT_PsmParCalc/3(TempStr)
  unit/1 -> ?
  ISP_wElec/1 -> Rate Transition2/1
  Rate Transition2/1 -> MCT_PsmParCalc/4(wElec)
  tempRotor/1 -> Saturation/1
  facFluxTemp_T/1 -> Product1/1
  psiExc_25degC/1 -> Product1/2
  Product1/1 -> MCT_PsmParCalc/5(PsiExcTemp)
  Saturation/1 -> facFluxTemp_T/1

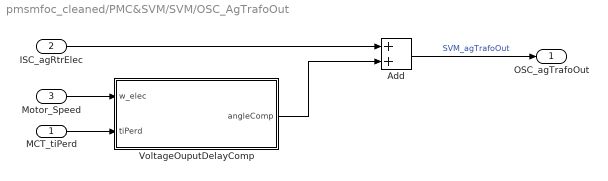
== system pmsmfoc_cleaned/PMC&SVM/SVM/OSC_AgTrafoOut ==
  MCT_tiPerd : Inport
  ISC_agRtrElec : Inport  Port=2
  Motor_Speed : Inport  Port=3
  Add : Sum  OutDataTypeStr=int16
  VoltageOuputDelayComp : MATLAB Function  TreatAsAtomicUnit=on
  OSC_agTrafoOut : Outport  VectorParamsAs1DForOutWhenUnconnected=off
  wires:
  Add/1 -> OSC_agTrafoOut/1  "SVM_agTrafoOut"
  ISC_agRtrElec/1 -> Add/1
  Motor_Speed/1 -> VoltageOuputDelayComp/1(w_elec)
  VoltageOuputDelayComp/1(angleComp) -> Add/2
  MCT_tiPerd/1 -> VoltageOuputDelayComp/2(tiPerd)

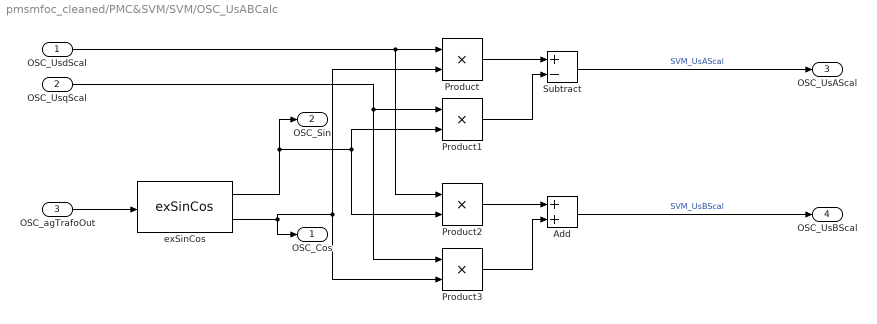
== system pmsmfoc_cleaned/PMC&SVM/SVM/OSC_UsABCalc ==
  OSC_UsdScal : Inport
  OSC_UsqScal : Inport  Port=2
  OSC_agTrafoOut : Inport  Port=3
  Add : Sum
  Product{,1..3} (4 alike) : Product  RndMeth=Zero
  Subtract : Sum  Inputs=+-
  exSinCos : MathLib/exSinCos
  OSC_Cos : Outport  VectorParamsAs1DForOutWhenUnconnected=off
  OSC_Sin : Outport  Port=2  VectorParamsAs1DForOutWhenUnconnected=off
  OSC_UsAScal : Outport  Port=3  VectorParamsAs1DForOutWhenUnconnected=off
  OSC_UsBScal : Outport  Port=4  VectorParamsAs1DForOutWhenUnconnected=off
  wires:
  OSC_agTrafoOut/1 -> exSinCos/1
  exSinCos/2 -> OSC_Cos/1, Product/2, Product3/2
  exSinCos/1 -> OSC_Sin/1, Product1/2, Product2/2
  Add/1 -> OSC_UsBScal/1  "SVM_UsBScal"
  Product3/1 -> Add/2
  Product2/1 -> Add/1
  OSC_UsqScal/1 -> Product3/1, Product1/1
  Subtract/1 -> OSC_UsAScal/1  "SVM_UsAScal"
  Product1/1 -> Subtract/2
  Product/1 -> Subtract/1
  OSC_UsdScal/1 -> Product2/1, Product/1

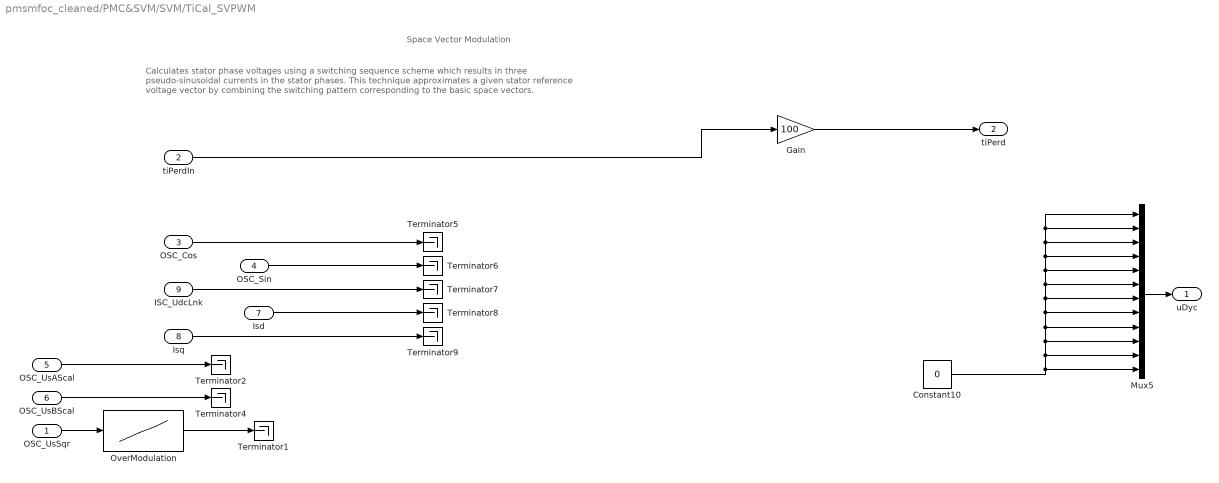
== system pmsmfoc_cleaned/PMC&SVM/SVM/TiCal_SVPWM ==
  note: Space Vector Modulation
  note: Calculates stator phase voltages using a switching sequence scheme which results in three pseudo-sinusoidal currents in the stator phases.
      | This technique approximates a given stator reference voltage vector by combining the switching pattern corresponding to the basic space vectors.
  OSC_UsSqr : Inport
  tiPerdIn : Inport  Port=2
  OSC_Cos : Inport  Port=3
  OSC_Sin : Inport  Port=4
  OSC_UsAScal : Inport  Port=5
  OSC_UsBScal : Inport  Port=6
  Isd : Inport  Port=7
  Isq : Inport  Port=8
  ISC_UdcLnk : Inport  Port=9
  Constant10 : Constant  Value=0
  Gain : Gain  Gain=100
      settings: AttributesFormatString=|
      | -------------------------
      | GTM clock 100MHz
  Mux5 : Mux  Inputs=12
  OverModulation : Lookup_n-D  NumberOfTableDimensions=1  BreakpointsForDimension1=[0 1 1.04 1.082 1.103 1.124 1.145 1.166 1.188 1.21 2]  BeginIndexSearchUsingPreviousIndexResult=on  Table="[1 1 1.05 1.15  1.22    1.31   1.45  1.68   4 10 10.0001]"  SampleTime=Tsw  InternalRulePriority=Speed  OutDataTypeStr=single
  Terminator{1..2,4..9} (8 alike) : Terminator
  uDyc : Outport  VectorParamsAs1DForOutWhenUnconnected=off
  tiPerd : Outport  Port=2  VectorParamsAs1DForOutWhenUnconnected=off
  wires:
  tiPerdIn/1 -> Gain/1
  Gain/1 -> tiPerd/1
  Mux5/1 -> uDyc/1
  OSC_Sin/1 -> Terminator6/1
  OSC_Cos/1 -> Terminator5/1
  OverModulation/1 -> Terminator1/1
  OSC_UsSqr/1 -> OverModulation/1
  OSC_UsAScal/1 -> Terminator2/1
  OSC_UsBScal/1 -> Terminator4/1
  ISC_UdcLnk/1 -> Terminator7/1
  Isd/1 -> Terminator8/1
  Isq/1 -> Terminator9/1
  Constant10/1 -> Mux5/12, Mux5/11, Mux5/10, Mux5/9, Mux5/8, Mux5/7, Mux5/6, Mux5/5, Mux5/4, Mux5/3, Mux5/2, Mux5/1

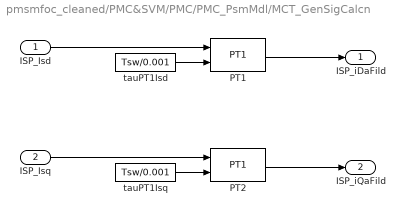
== system pmsmfoc_cleaned/PMC&SVM/PMC/PMC_PsmMdl/MCT_GenSigCalcn ==
  ISP_Isd : Inport  RequirementInfo={} %GIDa_ca7d1031_d465_4c92_a67c_0b7014c73c4c
  ISP_Isq : Inport  RequirementInfo={} %GIDa_abd2be4f_d8f0_4781_8926_cf7b1590379c  Port=2
  PT1 : MathLib/PT1  SystemSampleTime=-1  VariantActivationTime=update diagram  Latency=0  AutoFrameSizeCalculation=off
  PT2 : MathLib/PT1  SystemSampleTime=-1  VariantActivationTime=update diagram  Latency=0  AutoFrameSizeCalculation=off
  tauPT1Isd : Constant  RequirementInfo={} %GIDa_e050eea5_6865_433a_a2ac_897d3f186bef  Value=Tsw/0.001  OutDataTypeStr=single
  tauPT1Isq : Constant  RequirementInfo={} %GIDa_7e8f1d3b_0caa_4bb6_8994_f2b6a45655de  Value=Tsw/0.001  OutDataTypeStr=single
  ISP_iDaFild : Outport  RequirementInfo={} %GIDa_b55f899e_3979_404e_8e7e_ed1e12c13068  VectorParamsAs1DForOutWhenUnconnected=off
  ISP_iQaFild : Outport  RequirementInfo={} %GIDa_7bdf25e8_b1ec_4d26_aaee_23aded36c8c7  Port=2  VectorParamsAs1DForOutWhenUnconnected=off
  wires:
  ISP_Isq/1 -> PT2/1
  PT2/1 -> ISP_iQaFild/1
  tauPT1Isq/1 -> PT2/2
  ISP_Isd/1 -> PT1/1
  PT1/1 -> ISP_iDaFild/1
  tauPT1Isd/1 -> PT1/2
